simulink model "Mass_Matrix_Max_graphs_for_PID_params"  (R2019b)
settings: Solver=VariableStepAuto  StartTime=0.0  StopTime=10.0  RelTol=1e-3
libraries: dspmtrx3 x1, robotmaniplib x1
settings Model: Creator=PC  LastModifiedBy=PC

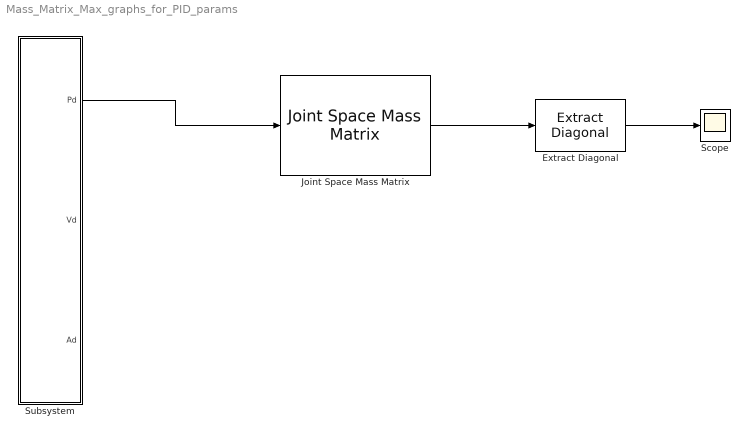
== system Mass_Matrix_Max_graphs_for_PID_params ==
  Extract Diagonal : dspmtrx3/Extract Diagonal
      settings: SourceProductName=DSP System Toolbox  SourceProductBaseCode=DS
  Joint Space Mass Matrix : robotmaniplib/Joint Space Mass Matrix  RigidBodyTree=robot  SimulateUsing=Interpreted execution
      settings: SourceProductName=Robotics System Toolbox
  Scope : Scope
  Subsystem : Subsystem
  wires:
  Subsystem/1("Pd ") -> Joint Space Mass Matrix/1
  Joint Space Mass Matrix/1 -> Extract Diagonal/1
  Extract Diagonal/1 -> Scope/1

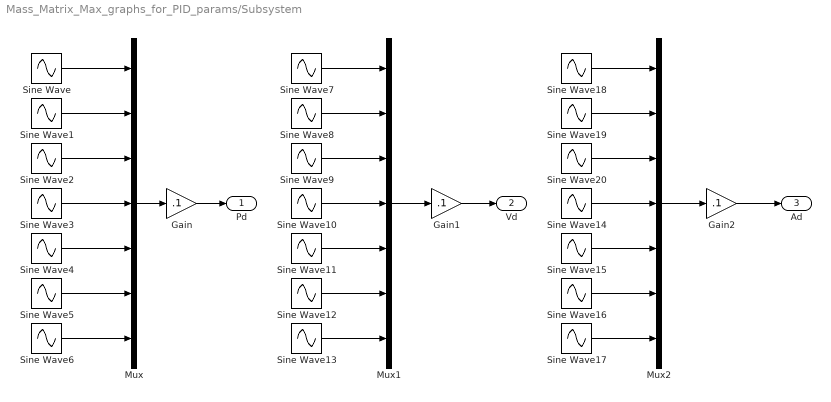
== system Mass_Matrix_Max_graphs_for_PID_params/Subsystem ==
  Gain : Gain  Gain=.1
  Gain1 : Gain  Gain=.1
  Gain2 : Gain  Gain=.1
  Mux : Mux  Inputs=7
  Mux1 : Mux  Inputs=7
  Mux2 : Mux  Inputs=7
  Sine Wave : Sin  Amplitude=7  SampleTime=0
  Sine Wave1 : Sin  Amplitude=6  SampleTime=0
  Sine Wave10 : Sin  Amplitude=4  Phase=pi/2  SampleTime=0
  Sine Wave11 : Sin  Amplitude=3  Phase=pi/2  SampleTime=0
  Sine Wave12 : Sin  Amplitude=2  Phase=pi/2  SampleTime=0
  Sine Wave13 : Sin  Phase=pi/2  SampleTime=0
  Sine Wave14 : Sin  Amplitude=4  Phase=pi  SampleTime=0
  Sine Wave15 : Sin  Amplitude=3  Phase=pi  SampleTime=0
  Sine Wave16 : Sin  Amplitude=2  Phase=pi  SampleTime=0
  Sine Wave17 : Sin  Phase=pi  SampleTime=0
  Sine Wave18 : Sin  Amplitude=7  Phase=pi  SampleTime=0
  Sine Wave19 : Sin  Amplitude=6  Phase=pi  SampleTime=0
  Sine Wave2 : Sin  Amplitude=5  SampleTime=0
  Sine Wave20 : Sin  Amplitude=5  Phase=pi  SampleTime=0
  Sine Wave3 : Sin  Amplitude=4  SampleTime=0
  Sine Wave4 : Sin  Amplitude=3  SampleTime=0
  Sine Wave5 : Sin  Amplitude=2  SampleTime=0
  Sine Wave6 : Sin  SampleTime=0
  Sine Wave7 : Sin  Amplitude=7  Phase=pi/2  SampleTime=0
  Sine Wave8 : Sin  Amplitude=6  Phase=pi/2  SampleTime=0
  Sine Wave9 : Sin  Amplitude=5  Phase=pi/2  SampleTime=0
  "Pd " : Outport  VectorParamsAs1DForOutWhenUnconnected=off
  "Vd " : Outport  Port=2  VectorParamsAs1DForOutWhenUnconnected=off
  "Ad " : Outport  Port=3  VectorParamsAs1DForOutWhenUnconnected=off
  wires:
  Sine Wave4/1 -> Mux/5
  Sine Wave5/1 -> Mux/6
  Sine Wave2/1 -> Mux/3
  Sine Wave/1 -> Mux/1
  Sine Wave6/1 -> Mux/7
  Sine Wave1/1 -> Mux/2
  Sine Wave3/1 -> Mux/4
  Mux/1 -> Gain/1
  Sine Wave10/1 -> Mux1/4
  Sine Wave9/1 -> Mux1/3
  Mux1/1 -> Gain1/1
  Sine Wave8/1 -> Mux1/2
  Sine Wave13/1 -> Mux1/7
  Sine Wave7/1 -> Mux1/1
  Sine Wave11/1 -> Mux1/5
  Sine Wave12/1 -> Mux1/6
  Sine Wave18/1 -> Mux2/1
  Sine Wave16/1 -> Mux2/6
  Sine Wave19/1 -> Mux2/2
  Sine Wave20/1 -> Mux2/3
  Sine Wave14/1 -> Mux2/4
  Mux2/1 -> Gain2/1
  Sine Wave17/1 -> Mux2/7
  Sine Wave15/1 -> Mux2/5
  Gain/1 -> "Pd "/1
  Gain1/1 -> "Vd "/1
  Gain2/1 -> "Ad "/1
